simulink model "dyn_nielin_mod_dyskretny"  (R2014b)
settings: Solver=ode45  StartTime=0.0  StopTime=tkonc  RelTol=1e-3
undefined symbols (not defined in the file or in its folder): a1, a2, a3, a4, K, T1, T2, Tp, x0
settings Model: Creator=Konrad  LastModifiedBy=Konrad

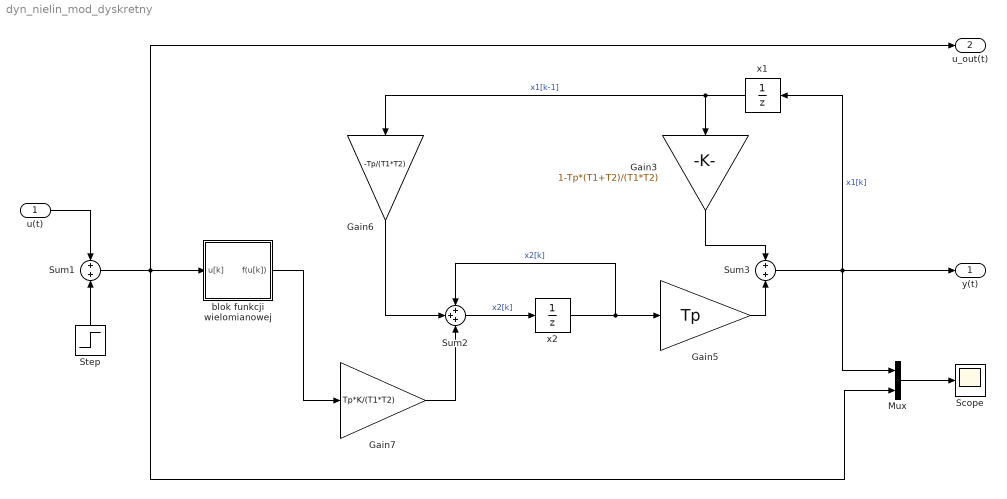
== system dyn_nielin_mod_dyskretny ==
  u(t) : Inport
  Gain3 : Gain  Gain=1-Tp*(T1+T2)/(T1*T2)
  Gain5 : Gain  Gain=Tp
  Gain6 : Gain  Gain=-Tp/(T1*T2)
  Gain7 : Gain  Gain=Tp*K/(T1*T2)
  Mux : Mux  Inputs=2
  Scope : Scope
  Step : Step  Time=step(1)  Before=step(2)  After=step(3)  SampleTime=0
  Sum1 : Sum  Inputs=+|+
  Sum2 : Sum  Inputs=+++
  Sum3 : Sum  Inputs=+|+
  blok funkcji wielomianowej : Subsystem
  x1 : UnitDelay  InitialCondition=x0(1)  SampleTime=Tp
  x2 : UnitDelay  InitialCondition=x0(2)  SampleTime=Tp
  y(t) : Outport
  u_out(t) : Outport  Port=2
  wires:
  Sum3/1 -> Mux/1, y(t)/1, x1/1  "x1[k]"
  Gain3/1 -> Sum3/1
  Gain5/1 -> Sum3/2
  Sum2/1 -> x2/1  "x2[k]"
  Gain6/1 -> Sum2/2
  blok funkcji wielomianowej/1(f(u[k])) -> Gain7/1
  Gain7/1 -> Sum2/3
  Mux/1 -> Scope/1
  x1/1 -> Gain3/1, Gain6/1  "x1[k-1]"
  x2/1 -> Gain5/1, Sum2/1  "x2[k]"
  Sum1/1 -> u_out(t)/1, blok funkcji wielomianowej/1(u[k]), Mux/2
  Step/1 -> Sum1/2
  u(t)/1 -> Sum1/1

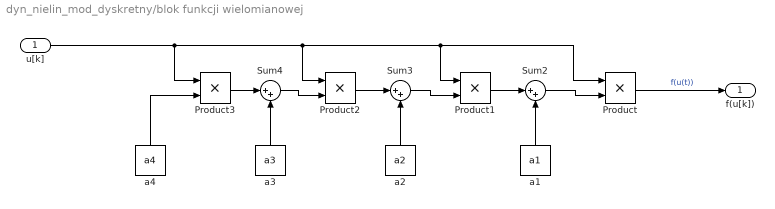
== system dyn_nielin_mod_dyskretny/blok funkcji wielomianowej ==
  u[k] : Inport
  Product{,1..3} (4 alike) : Product
  Sum2 : Sum  Inputs=|++
  Sum3 : Sum  Inputs=|++
  Sum4 : Sum  Inputs=|++
  a1 : Constant  Value=a1
  a2 : Constant  Value=a2
  a3 : Constant  Value=a3
  a4 : Constant  Value=a4
  f(u[k]) : Outport
  wires:
  u[k]/1 -> Product/1, Product1/1, Product2/1, Product3/1
  Product1/1 -> Sum2/1
  Product2/1 -> Sum3/1
  Sum2/1 -> Product/2
  Product/1 -> f(u[k])/1  "f(u(t))"
  Product3/1 -> Sum4/1
  a1/1 -> Sum2/2
  a2/1 -> Sum3/2
  Sum3/1 -> Product1/2
  a3/1 -> Sum4/2
  Sum4/1 -> Product2/2
  a4/1 -> Product3/2
